simulink model "sinewave1phaseto3phaseinverter"  (R2020a)
settings: Solver=VariableStepAuto  StartTime=0.0  StopTime=.5  RelTol=1e-3
libraries: powerlib x56, simulink x3, powerlib_meascontrol x3
settings Model: Creator=hp  LastModifiedBy=hp

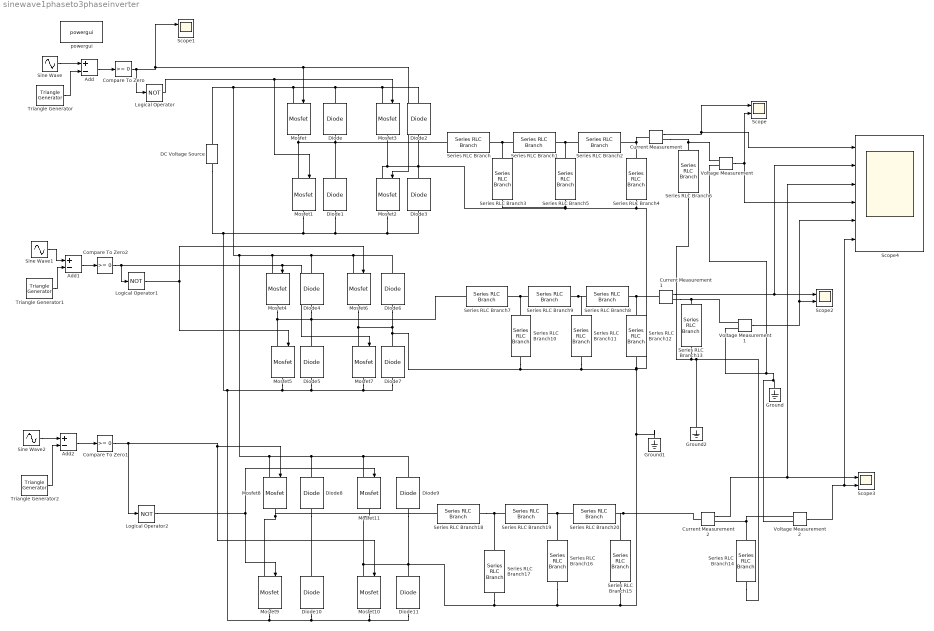
== system sinewave1phaseto3phaseinverter ==
  Add : Sum  Inputs=+-
  Add1 : Sum  Inputs=+-
  Add2 : Sum  Inputs=+-
  Compare To Zero : simulink/Logic and Bit Operations/Compare To Zero  relop=>=  OutDataTypeStr=boolean
  Compare To Zero1 : simulink/Logic and Bit Operations/Compare To Zero  relop=>=  OutDataTypeStr=boolean
  Compare To Zero2 : simulink/Logic and Bit Operations/Compare To Zero  relop=>=  OutDataTypeStr=boolean
  Current Measurement : powerlib/Measurements/Current Measurement  PhasorSimulation=off  OutputType=Complex  PSBequivalent=0
  Current Measurement1 : powerlib/Measurements/Current Measurement  PhasorSimulation=off  OutputType=Complex  PSBequivalent=0
  Current Measurement2 : powerlib/Measurements/Current Measurement  PhasorSimulation=off  OutputType=Complex  PSBequivalent=0
  DC Voltage Source : powerlib/Electrical Sources/DC Voltage Source  Amplitude=100  Measurements=None
  Diode{,1..11} (12 alike) : powerlib/Power Electronics/Diode  Ron=0.001  Lon=0  Vf=0.8  IC=0  UseSnubber=0  Rs=500  Cs=250e-9  Measurements=off
  Ground : powerlib/Elements/Ground  LConnTagsString=a
  Ground1 : powerlib/Elements/Ground  LConnTagsString=a
  Ground2 : powerlib/Elements/Ground  LConnTagsString=a
  Logical Operator : Logic  Operator=NOT  AllPortsSameDT=off  OutDataTypeStr=boolean
  Logical Operator1 : Logic  Operator=NOT  AllPortsSameDT=off  OutDataTypeStr=boolean
  Logical Operator2 : Logic  Operator=NOT  AllPortsSameDT=off  OutDataTypeStr=boolean
  Mosfet{,1..11} (12 alike) : powerlib/Power Electronics/Mosfet  Ron=0.1  Lon=0  Rd=0.01  Vfd=0  IC=0  Rs=1e5  Cs=inf  Measurements=off
  Scope{,1..3} (4 alike) : Scope  NumInputPorts=2
  Scope4 : Scope  NumInputPorts=6
  Series RLC Branch{,1..2,7..9,18..20} (9 alike) : powerlib/Elements/Series RLC Branch  LConnTagsString=__new0  RConnTagsString=__new0  BranchType=R  Resistance=1  Inductance=1e-3  SetiL0=off  InitialCurrent=0  Capacitance=1e-6  Setx0=off  InitialVoltage=0  Measurements=None
  Series RLC Branch{3..5,10..12,15..17} (9 alike) : powerlib/Elements/Series RLC Branch  LConnTagsString=__new0  RConnTagsString=__new0  BranchType=C  Resistance=1  Inductance=1e-3  SetiL0=off  InitialCurrent=0  Capacitance=3.18e-3  Setx0=off  InitialVoltage=0  Measurements=None
  Series RLC Branch13 : powerlib/Elements/Series RLC Branch  LConnTagsString=__new0  RConnTagsString=__new0  BranchType=R  Resistance=10  Inductance=1e-3  SetiL0=off  InitialCurrent=0  Capacitance=1e-6  Setx0=off  InitialVoltage=0  Measurements=None
  Series RLC Branch14 : powerlib/Elements/Series RLC Branch  LConnTagsString=__new0  RConnTagsString=__new0  BranchType=R  Resistance=10  Inductance=1e-3  SetiL0=off  InitialCurrent=0  Capacitance=1e-6  Setx0=off  InitialVoltage=0  Measurements=None
  Series RLC Branch6 : powerlib/Elements/Series RLC Branch  LConnTagsString=__new0  RConnTagsString=__new0  BranchType=R  Resistance=10  Inductance=1e-3  SetiL0=off  InitialCurrent=0  Capacitance=1e-6  Setx0=off  InitialVoltage=0  Measurements=None
  Sine Wave : Sin  Amplitude=20  Frequency=2*pi*50  SampleTime=0
  Sine Wave1 : Sin  Amplitude=20  Frequency=2*pi*50  Phase=120*pi/180  SampleTime=0
  Sine Wave2 : Sin  Amplitude=20  Frequency=2*pi*50  Phase=240*pi/180  SampleTime=0
  Triangle Generator : powerlib_meascontrol/Pulse & Signal Generators/Triangle Generator  Freq=1000  Phase=90  Ts=0
  Triangle Generator1 : powerlib_meascontrol/Pulse & Signal Generators/Triangle Generator  Freq=1000  Phase=90  Ts=0
  Triangle Generator2 : powerlib_meascontrol/Pulse & Signal Generators/Triangle Generator  Freq=1e3  Phase=90  Ts=0
  Voltage Measurement : powerlib/Measurements/Voltage Measurement  PhasorSimulation=off  OutputType=Complex  PSBequivalent=0
  Voltage Measurement1 : powerlib/Measurements/Voltage Measurement  PhasorSimulation=off  OutputType=Complex  PSBequivalent=0
  Voltage Measurement2 : powerlib/Measurements/Voltage Measurement  PhasorSimulation=off  OutputType=Complex  PSBequivalent=0
  powergui : powerlib/powergui  Priority=1  SimulationMode=Discrete  SampleTime=50e-6  frequency=60  Iterations=50  frequencyindice=0  Pbase=100e6  ErrMax=1e-4  UnitsV=kV  UnitsW=MW  buscounter=0  FunctionMessages=off  echomessages=off  EnableUseOfTLC=off  CurrentSourceSwitches=off  DisableSnubberDevices=off  DisableRonSwitches=off  DisableVfSwitches=off  DisplayEquations=off  AutomaticDiscreteSolvers=off  SolverType=Tustin/Backward Euler (TBE)  Interpol=off  ExternalGateDelay=off  methode=off  Ts=100  x0status=blocks  SPID=on  SwTol=0  HookPort=off  NonlinearTolerance=1e-4  nMaxIteration=100  ContinueOnMaxIteration=off  RestoreLinks=warning  ResistiveCurrentMeasurement=off  Frange=[0:2:500]  Ylog=off  Xlog=on  ShowGrid=off  save=off  variable=ZData  structure=0  ZoomFFT=off  StartTime=0.0  cycles=1  DisplayStyle=1  fundamental=60  FreqAxis=off  MaxFrequency=1000  frequencyindicesteady=1  RmsSteady=1  display=off
  wires:
  Sine Wave/1 -> Add/1
  Triangle Generator/1 -> Add/2
  Add/1 -> Compare To Zero/1
  Add1/1 -> Compare To Zero2/1
  Sine Wave1/1 -> Add1/1
  Triangle Generator1/1 -> Add1/2
  Sine Wave2/1 -> Add2/1
  Triangle Generator2/1 -> Add2/2
  Add2/1 -> Compare To Zero1/1
  Compare To Zero2/1 -> Mosfet7/1, Mosfet4/1, Logical Operator1/1
  Compare To Zero1/1 -> Mosfet10/1, Mosfet8/1, Logical Operator2/1
  Voltage Measurement/1 -> Scope4/4, Scope/2
  Compare To Zero/1 -> Mosfet2/1, Mosfet/1, Scope1/1, Logical Operator/1
  Logical Operator/1 -> Mosfet1/1, Mosfet3/1
  Logical Operator1/1 -> Mosfet6/1, Mosfet5/1
  Logical Operator2/1 -> Mosfet9/1, Mosfet11/1
  Voltage Measurement2/1 -> Scope4/6, Scope3/2
  Current Measurement2/1 -> Scope4/3, Scope3/1
  Voltage Measurement1/1 -> Scope4/5, Scope2/2
  Current Measurement1/1 -> Scope4/2, Scope2/1
  Current Measurement/1 -> Scope4/1, Scope/1
  connections:
  Series RLC Branch1/LConn1 -- Series RLC Branch3/LConn1 -- Series RLC Branch/RConn1
  Series RLC Branch2/LConn1 -- Series RLC Branch5/LConn1 -- Series RLC Branch1/RConn1
  Series RLC Branch4/LConn1 -- Current Measurement/LConn1 -- Series RLC Branch2/RConn1
  Series RLC Branch15/RConn1 -- Ground1/LConn1 -- Series RLC Branch3/RConn1 -- Series RLC Branch5/RConn1 -- Diode3/RConn1 -- Mosfet2/LConn1 -- Mosfet3/RConn1 -- Diode2/LConn1 -- Series RLC Branch4/RConn1 -- Series RLC Branch12/RConn1 -- Diode6/LConn1 -- Mosfet7/LConn1 -- Mosfet6/RConn1 -- Diode7/RConn1 -- Series RLC Branch10/RConn1 -- Series RLC Branch11/RConn1 -- Series RLC Branch16/RConn1 -- Series RLC Branch17/RConn1 -- Mosfet11/RConn1 -- Mosfet10/LConn1 -- Diode9/LConn1 -- Diode11/RConn1
  DC Voltage Source/RConn1 -- Mosfet11/LConn1 -- Diode9/RConn1 -- Diode8/RConn1 -- Mosfet8/LConn1 -- Mosfet6/LConn1 -- Diode6/RConn1 -- Diode4/RConn1 -- Mosfet4/LConn1 -- Mosfet3/LConn1 -- Diode2/RConn1 -- Diode/RConn1 -- Mosfet/LConn1
  DC Voltage Source/LConn1 -- Diode11/LConn1 -- Mosfet10/RConn1 -- Diode10/LConn1 -- Mosfet9/RConn1 -- Diode7/LConn1 -- Mosfet7/RConn1 -- Diode5/LConn1 -- Mosfet5/RConn1 -- Mosfet1/RConn1 -- Diode3/LConn1 -- Mosfet2/RConn1 -- Diode1/LConn1
  Mosfet/RConn1 -- Series RLC Branch/LConn1 -- Diode1/RConn1 -- Diode/LConn1 -- Mosfet1/LConn1
  Series RLC Branch6/LConn1 -- Current Measurement/RConn1 -- Voltage Measurement/LConn1
  Series RLC Branch9/LConn1 -- Series RLC Branch10/LConn1 -- Series RLC Branch7/RConn1
  Series RLC Branch8/LConn1 -- Series RLC Branch11/LConn1 -- Series RLC Branch9/RConn1
  Series RLC Branch12/LConn1 -- Current Measurement1/LConn1 -- Series RLC Branch8/RConn1
  Series RLC Branch7/LConn1 -- Diode4/LConn1 -- Diode5/RConn1 -- Mosfet5/LConn1 -- Mosfet4/RConn1
  Current Measurement1/RConn1 -- Voltage Measurement1/LConn1 -- Series RLC Branch13/LConn1
  Series RLC Branch20/LConn1 -- Series RLC Branch16/LConn1 -- Series RLC Branch19/RConn1
  Series RLC Branch18/RConn1 -- Series RLC Branch17/LConn1 -- Series RLC Branch19/LConn1
  Current Measurement2/LConn1 -- Series RLC Branch15/LConn1 -- Series RLC Branch20/RConn1
  Series RLC Branch18/LConn1 -- Mosfet9/LConn1 -- Mosfet8/RConn1
  Diode8/LConn1 -- Diode10/RConn1
  Series RLC Branch14/LConn1 -- Voltage Measurement2/LConn1 -- Current Measurement2/RConn1
  Series RLC Branch6/RConn1 -- Ground2/LConn1 -- Series RLC Branch14/RConn1 -- Series RLC Branch13/RConn1
  Ground/LConn1 -- Voltage Measurement/LConn2 -- Voltage Measurement1/LConn2 -- Voltage Measurement2/LConn2
